simulink model "modificar_acc_compilar"  (R2013b)
settings: Solver=ode45  StartTime=0.0  StopTime=17000  RelTol=1e-3
undefined symbols (not defined in the file): internal_oor, misc_lib, pfb_coeff_gen_calc, xlfda_numerator, xlipgetpartsetting
libraries: xbsIndex_r4 x1539, xps_library x14, dspsigops x8, casper_library_misc x8, casper_library_delays x3, simulink x1
(part 3 of 15)

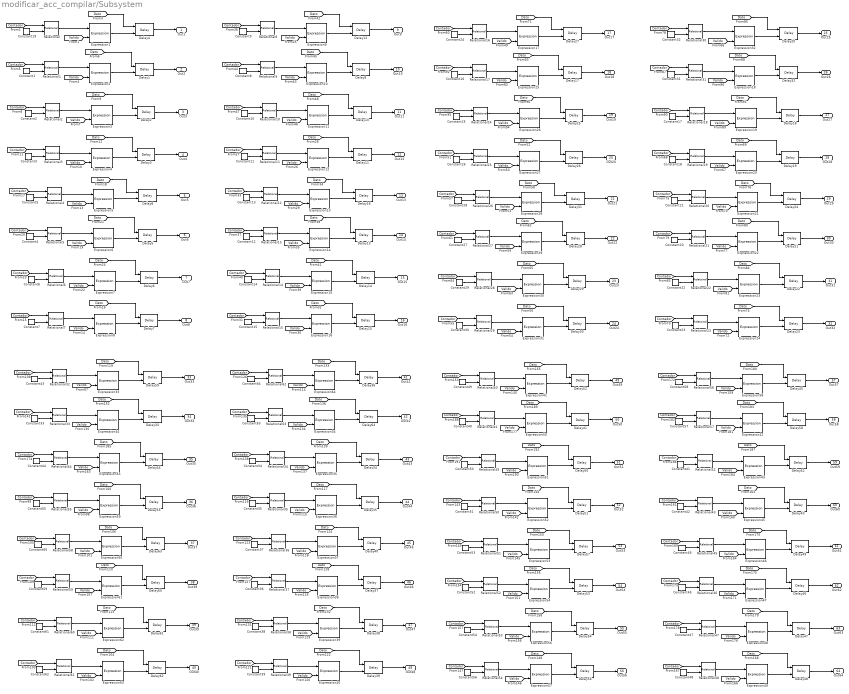
== system modificar_acc_compilar/Subsystem ==
  Constant1 : xbsIndex_r4/Constant  const=1  gui_display_data_type=Fixed-point  arith_type=Unsigned  n_bits=6  bin_pt=0  preci_type=Single  exp_width=8  frac_width=24  explicit_period=on  period=1  equ=P=C  opselect=C  inp2=PCIN>>17  opr=+  inp1=P  carry=CIN  dbl_ovrd=off  block_type=constant
  Constant10 : xbsIndex_r4/Constant  const=10  gui_display_data_type=Fixed-point  arith_type=Unsigned  n_bits=6  bin_pt=0  preci_type=Single  exp_width=8  frac_width=24  explicit_period=on  period=1  equ=P=C  opselect=C  inp2=PCIN>>17  opr=+  inp1=P  carry=CIN  dbl_ovrd=off  block_type=constant
  Constant11 : xbsIndex_r4/Constant  const=11  gui_display_data_type=Fixed-point  arith_type=Unsigned  n_bits=6  bin_pt=0  preci_type=Single  exp_width=8  frac_width=24  explicit_period=on  period=1  equ=P=C  opselect=C  inp2=PCIN>>17  opr=+  inp1=P  carry=CIN  dbl_ovrd=off  block_type=constant
  Constant12 : xbsIndex_r4/Constant  const=13  gui_display_data_type=Fixed-point  arith_type=Unsigned  n_bits=6  bin_pt=0  preci_type=Single  exp_width=8  frac_width=24  explicit_period=on  period=1  equ=P=C  opselect=C  inp2=PCIN>>17  opr=+  inp1=P  carry=CIN  dbl_ovrd=off  block_type=constant
  Constant13 : xbsIndex_r4/Constant  const=12  gui_display_data_type=Fixed-point  arith_type=Unsigned  n_bits=6  bin_pt=0  preci_type=Single  exp_width=8  frac_width=24  explicit_period=on  period=1  equ=P=C  opselect=C  inp2=PCIN>>17  opr=+  inp1=P  carry=CIN  dbl_ovrd=off  block_type=constant
  Constant14 : xbsIndex_r4/Constant  const=14  gui_display_data_type=Fixed-point  arith_type=Unsigned  n_bits=6  bin_pt=0  preci_type=Single  exp_width=8  frac_width=24  explicit_period=on  period=1  equ=P=C  opselect=C  inp2=PCIN>>17  opr=+  inp1=P  carry=CIN  dbl_ovrd=off  block_type=constant
  Constant15 : xbsIndex_r4/Constant  const=15  gui_display_data_type=Fixed-point  arith_type=Unsigned  n_bits=6  bin_pt=0  preci_type=Single  exp_width=8  frac_width=24  explicit_period=on  period=1  equ=P=C  opselect=C  inp2=PCIN>>17  opr=+  inp1=P  carry=CIN  dbl_ovrd=off  block_type=constant
  Constant16 : xbsIndex_r4/Constant  const=17  gui_display_data_type=Fixed-point  arith_type=Unsigned  n_bits=6  bin_pt=0  preci_type=Single  exp_width=8  frac_width=24  explicit_period=on  period=1  equ=P=C  opselect=C  inp2=PCIN>>17  opr=+  inp1=P  carry=CIN  dbl_ovrd=off  block_type=constant
  Constant17 : xbsIndex_r4/Constant  const=26  gui_display_data_type=Fixed-point  arith_type=Unsigned  n_bits=6  bin_pt=0  preci_type=Single  exp_width=8  frac_width=24  explicit_period=on  period=1  equ=P=C  opselect=C  inp2=PCIN>>17  opr=+  inp1=P  carry=CIN  dbl_ovrd=off  block_type=constant
  Constant18 : xbsIndex_r4/Constant  const=27  gui_display_data_type=Fixed-point  arith_type=Unsigned  n_bits=6  bin_pt=0  preci_type=Single  exp_width=8  frac_width=24  explicit_period=on  period=1  equ=P=C  opselect=C  inp2=PCIN>>17  opr=+  inp1=P  carry=CIN  dbl_ovrd=off  block_type=constant
  Constant19 : xbsIndex_r4/Constant  const=0  gui_display_data_type=Fixed-point  arith_type=Unsigned  n_bits=6  bin_pt=0  preci_type=Single  exp_width=8  frac_width=24  explicit_period=on  period=1  equ=P=C  opselect=C  inp2=PCIN>>17  opr=+  inp1=P  carry=CIN  dbl_ovrd=off  block_type=constant
  Constant2 : xbsIndex_r4/Constant  const=2  gui_display_data_type=Fixed-point  arith_type=Unsigned  n_bits=6  bin_pt=0  preci_type=Single  exp_width=8  frac_width=24  explicit_period=on  period=1  equ=P=C  opselect=C  inp2=PCIN>>17  opr=+  inp1=P  carry=CIN  dbl_ovrd=off  block_type=constant
  Constant20 : xbsIndex_r4/Constant  const=29  gui_display_data_type=Fixed-point  arith_type=Unsigned  n_bits=6  bin_pt=0  preci_type=Single  exp_width=8  frac_width=24  explicit_period=on  period=1  equ=P=C  opselect=C  inp2=PCIN>>17  opr=+  inp1=P  carry=CIN  dbl_ovrd=off  block_type=constant
  Constant21 : xbsIndex_r4/Constant  const=28  gui_display_data_type=Fixed-point  arith_type=Unsigned  n_bits=6  bin_pt=0  preci_type=Single  exp_width=8  frac_width=24  explicit_period=on  period=1  equ=P=C  opselect=C  inp2=PCIN>>17  opr=+  inp1=P  carry=CIN  dbl_ovrd=off  block_type=constant
  Constant22 : xbsIndex_r4/Constant  const=30  gui_display_data_type=Fixed-point  arith_type=Unsigned  n_bits=6  bin_pt=0  preci_type=Single  exp_width=8  frac_width=24  explicit_period=on  period=1  equ=P=C  opselect=C  inp2=PCIN>>17  opr=+  inp1=P  carry=CIN  dbl_ovrd=off  block_type=constant
  Constant23 : xbsIndex_r4/Constant  const=31  gui_display_data_type=Fixed-point  arith_type=Unsigned  n_bits=6  bin_pt=0  preci_type=Single  exp_width=8  frac_width=24  explicit_period=on  period=1  equ=P=C  opselect=C  inp2=PCIN>>17  opr=+  inp1=P  carry=CIN  dbl_ovrd=off  block_type=constant
  Constant24 : xbsIndex_r4/Constant  const=16  gui_display_data_type=Fixed-point  arith_type=Unsigned  n_bits=6  bin_pt=0  preci_type=Single  exp_width=8  frac_width=24  explicit_period=on  period=1  equ=P=C  opselect=C  inp2=PCIN>>17  opr=+  inp1=P  carry=CIN  dbl_ovrd=off  block_type=constant
  Constant25 : xbsIndex_r4/Constant  const=18  gui_display_data_type=Fixed-point  arith_type=Unsigned  n_bits=6  bin_pt=0  preci_type=Single  exp_width=8  frac_width=24  explicit_period=on  period=1  equ=P=C  opselect=C  inp2=PCIN>>17  opr=+  inp1=P  carry=CIN  dbl_ovrd=off  block_type=constant
  Constant26 : xbsIndex_r4/Constant  const=19  gui_display_data_type=Fixed-point  arith_type=Unsigned  n_bits=6  bin_pt=0  preci_type=Single  exp_width=8  frac_width=24  explicit_period=on  period=1  equ=P=C  opselect=C  inp2=PCIN>>17  opr=+  inp1=P  carry=CIN  dbl_ovrd=off  block_type=constant
  Constant27 : xbsIndex_r4/Constant  const=21  gui_display_data_type=Fixed-point  arith_type=Unsigned  n_bits=6  bin_pt=0  preci_type=Single  exp_width=8  frac_width=24  explicit_period=on  period=1  equ=P=C  opselect=C  inp2=PCIN>>17  opr=+  inp1=P  carry=CIN  dbl_ovrd=off  block_type=constant
  Constant28 : xbsIndex_r4/Constant  const=20  gui_display_data_type=Fixed-point  arith_type=Unsigned  n_bits=6  bin_pt=0  preci_type=Single  exp_width=8  frac_width=24  explicit_period=on  period=1  equ=P=C  opselect=C  inp2=PCIN>>17  opr=+  inp1=P  carry=CIN  dbl_ovrd=off  block_type=constant
  Constant29 : xbsIndex_r4/Constant  const=22  gui_display_data_type=Fixed-point  arith_type=Unsigned  n_bits=6  bin_pt=0  preci_type=Single  exp_width=8  frac_width=24  explicit_period=on  period=1  equ=P=C  opselect=C  inp2=PCIN>>17  opr=+  inp1=P  carry=CIN  dbl_ovrd=off  block_type=constant
  Constant3 : xbsIndex_r4/Constant  const=3  gui_display_data_type=Fixed-point  arith_type=Unsigned  n_bits=6  bin_pt=0  preci_type=Single  exp_width=8  frac_width=24  explicit_period=on  period=1  equ=P=C  opselect=C  inp2=PCIN>>17  opr=+  inp1=P  carry=CIN  dbl_ovrd=off  block_type=constant
  Constant30 : xbsIndex_r4/Constant  const=23  gui_display_data_type=Fixed-point  arith_type=Unsigned  n_bits=6  bin_pt=0  preci_type=Single  exp_width=8  frac_width=24  explicit_period=on  period=1  equ=P=C  opselect=C  inp2=PCIN>>17  opr=+  inp1=P  carry=CIN  dbl_ovrd=off  block_type=constant
  Constant31 : xbsIndex_r4/Constant  const=25  gui_display_data_type=Fixed-point  arith_type=Unsigned  n_bits=6  bin_pt=0  preci_type=Single  exp_width=8  frac_width=24  explicit_period=on  period=1  equ=P=C  opselect=C  inp2=PCIN>>17  opr=+  inp1=P  carry=CIN  dbl_ovrd=off  block_type=constant
  Constant32 : xbsIndex_r4/Constant  const=24  gui_display_data_type=Fixed-point  arith_type=Unsigned  n_bits=6  bin_pt=0  preci_type=Single  exp_width=8  frac_width=24  explicit_period=on  period=1  equ=P=C  opselect=C  inp2=PCIN>>17  opr=+  inp1=P  carry=CIN  dbl_ovrd=off  block_type=constant
  Constant33 : xbsIndex_r4/Constant  const=33  gui_display_data_type=Fixed-point  arith_type=Unsigned  n_bits=6  bin_pt=0  preci_type=Single  exp_width=8  frac_width=24  explicit_period=on  period=1  equ=P=C  opselect=C  inp2=PCIN>>17  opr=+  inp1=P  carry=CIN  dbl_ovrd=off  block_type=constant
  Constant34 : xbsIndex_r4/Constant  const=42  gui_display_data_type=Fixed-point  arith_type=Unsigned  n_bits=6  bin_pt=0  preci_type=Single  exp_width=8  frac_width=24  explicit_period=on  period=1  equ=P=C  opselect=C  inp2=PCIN>>17  opr=+  inp1=P  carry=CIN  dbl_ovrd=off  block_type=constant
  Constant35 : xbsIndex_r4/Constant  const=43  gui_display_data_type=Fixed-point  arith_type=Unsigned  n_bits=6  bin_pt=0  preci_type=Single  exp_width=8  frac_width=24  explicit_period=on  period=1  equ=P=C  opselect=C  inp2=PCIN>>17  opr=+  inp1=P  carry=CIN  dbl_ovrd=off  block_type=constant
  Constant36 : xbsIndex_r4/Constant  const=45  gui_display_data_type=Fixed-point  arith_type=Unsigned  n_bits=6  bin_pt=0  preci_type=Single  exp_width=8  frac_width=24  explicit_period=on  period=1  equ=P=C  opselect=C  inp2=PCIN>>17  opr=+  inp1=P  carry=CIN  dbl_ovrd=off  block_type=constant
  Constant37 : xbsIndex_r4/Constant  const=44  gui_display_data_type=Fixed-point  arith_type=Unsigned  n_bits=6  bin_pt=0  preci_type=Single  exp_width=8  frac_width=24  explicit_period=on  period=1  equ=P=C  opselect=C  inp2=PCIN>>17  opr=+  inp1=P  carry=CIN  dbl_ovrd=off  block_type=constant
  Constant38 : xbsIndex_r4/Constant  const=46  gui_display_data_type=Fixed-point  arith_type=Unsigned  n_bits=6  bin_pt=0  preci_type=Single  exp_width=8  frac_width=24  explicit_period=on  period=1  equ=P=C  opselect=C  inp2=PCIN>>17  opr=+  inp1=P  carry=CIN  dbl_ovrd=off  block_type=constant
  Constant39 : xbsIndex_r4/Constant  const=47  gui_display_data_type=Fixed-point  arith_type=Unsigned  n_bits=6  bin_pt=0  preci_type=Single  exp_width=8  frac_width=24  explicit_period=on  period=1  equ=P=C  opselect=C  inp2=PCIN>>17  opr=+  inp1=P  carry=CIN  dbl_ovrd=off  block_type=constant
  Constant4 : xbsIndex_r4/Constant  const=5  gui_display_data_type=Fixed-point  arith_type=Unsigned  n_bits=6  bin_pt=0  preci_type=Single  exp_width=8  frac_width=24  explicit_period=on  period=1  equ=P=C  opselect=C  inp2=PCIN>>17  opr=+  inp1=P  carry=CIN  dbl_ovrd=off  block_type=constant
  Constant40 : xbsIndex_r4/Constant  const=49  gui_display_data_type=Fixed-point  arith_type=Unsigned  n_bits=6  bin_pt=0  preci_type=Single  exp_width=8  frac_width=24  explicit_period=on  period=1  equ=P=C  opselect=C  inp2=PCIN>>17  opr=+  inp1=P  carry=CIN  dbl_ovrd=off  block_type=constant
  Constant41 : xbsIndex_r4/Constant  const=58  gui_display_data_type=Fixed-point  arith_type=Unsigned  n_bits=6  bin_pt=0  preci_type=Single  exp_width=8  frac_width=24  explicit_period=on  period=1  equ=P=C  opselect=C  inp2=PCIN>>17  opr=+  inp1=P  carry=CIN  dbl_ovrd=off  block_type=constant
  Constant42 : xbsIndex_r4/Constant  const=59  gui_display_data_type=Fixed-point  arith_type=Unsigned  n_bits=6  bin_pt=0  preci_type=Single  exp_width=8  frac_width=24  explicit_period=on  period=1  equ=P=C  opselect=C  inp2=PCIN>>17  opr=+  inp1=P  carry=CIN  dbl_ovrd=off  block_type=constant
  Constant43 : xbsIndex_r4/Constant  const=32  gui_display_data_type=Fixed-point  arith_type=Unsigned  n_bits=6  bin_pt=0  preci_type=Single  exp_width=8  frac_width=24  explicit_period=on  period=1  equ=P=C  opselect=C  inp2=PCIN>>17  opr=+  inp1=P  carry=CIN  dbl_ovrd=off  block_type=constant
  Constant44 : xbsIndex_r4/Constant  const=34  gui_display_data_type=Fixed-point  arith_type=Unsigned  n_bits=6  bin_pt=0  preci_type=Single  exp_width=8  frac_width=24  explicit_period=on  period=1  equ=P=C  opselect=C  inp2=PCIN>>17  opr=+  inp1=P  carry=CIN  dbl_ovrd=off  block_type=constant
  Constant45 : xbsIndex_r4/Constant  const=61  gui_display_data_type=Fixed-point  arith_type=Unsigned  n_bits=6  bin_pt=0  preci_type=Single  exp_width=8  frac_width=24  explicit_period=on  period=1  equ=P=C  opselect=C  inp2=PCIN>>17  opr=+  inp1=P  carry=CIN  dbl_ovrd=off  block_type=constant
  Constant46 : xbsIndex_r4/Constant  const=60  gui_display_data_type=Fixed-point  arith_type=Unsigned  n_bits=6  bin_pt=0  preci_type=Single  exp_width=8  frac_width=24  explicit_period=on  period=1  equ=P=C  opselect=C  inp2=PCIN>>17  opr=+  inp1=P  carry=CIN  dbl_ovrd=off  block_type=constant
  Constant47 : xbsIndex_r4/Constant  const=62  gui_display_data_type=Fixed-point  arith_type=Unsigned  n_bits=6  bin_pt=0  preci_type=Single  exp_width=8  frac_width=24  explicit_period=on  period=1  equ=P=C  opselect=C  inp2=PCIN>>17  opr=+  inp1=P  carry=CIN  dbl_ovrd=off  block_type=constant
  Constant48 : xbsIndex_r4/Constant  const=63  gui_display_data_type=Fixed-point  arith_type=Unsigned  n_bits=6  bin_pt=0  preci_type=Single  exp_width=8  frac_width=24  explicit_period=on  period=1  equ=P=C  opselect=C  inp2=PCIN>>17  opr=+  inp1=P  carry=CIN  dbl_ovrd=off  block_type=constant
  Constant49 : xbsIndex_r4/Constant  const=48  gui_display_data_type=Fixed-point  arith_type=Unsigned  n_bits=6  bin_pt=0  preci_type=Single  exp_width=8  frac_width=24  explicit_period=on  period=1  equ=P=C  opselect=C  inp2=PCIN>>17  opr=+  inp1=P  carry=CIN  dbl_ovrd=off  block_type=constant
  Constant5 : xbsIndex_r4/Constant  const=4  gui_display_data_type=Fixed-point  arith_type=Unsigned  n_bits=6  bin_pt=0  preci_type=Single  exp_width=8  frac_width=24  explicit_period=on  period=1  equ=P=C  opselect=C  inp2=PCIN>>17  opr=+  inp1=P  carry=CIN  dbl_ovrd=off  block_type=constant
  Constant50 : xbsIndex_r4/Constant  const=50  gui_display_data_type=Fixed-point  arith_type=Unsigned  n_bits=6  bin_pt=0  preci_type=Single  exp_width=8  frac_width=24  explicit_period=on  period=1  equ=P=C  opselect=C  inp2=PCIN>>17  opr=+  inp1=P  carry=CIN  dbl_ovrd=off  block_type=constant
  Constant51 : xbsIndex_r4/Constant  const=51  gui_display_data_type=Fixed-point  arith_type=Unsigned  n_bits=6  bin_pt=0  preci_type=Single  exp_width=8  frac_width=24  explicit_period=on  period=1  equ=P=C  opselect=C  inp2=PCIN>>17  opr=+  inp1=P  carry=CIN  dbl_ovrd=off  block_type=constant
  Constant52 : xbsIndex_r4/Constant  const=53  gui_display_data_type=Fixed-point  arith_type=Unsigned  n_bits=6  bin_pt=0  preci_type=Single  exp_width=8  frac_width=24  explicit_period=on  period=1  equ=P=C  opselect=C  inp2=PCIN>>17  opr=+  inp1=P  carry=CIN  dbl_ovrd=off  block_type=constant
  Constant53 : xbsIndex_r4/Constant  const=52  gui_display_data_type=Fixed-point  arith_type=Unsigned  n_bits=6  bin_pt=0  preci_type=Single  exp_width=8  frac_width=24  explicit_period=on  period=1  equ=P=C  opselect=C  inp2=PCIN>>17  opr=+  inp1=P  carry=CIN  dbl_ovrd=off  block_type=constant
  Constant54 : xbsIndex_r4/Constant  const=54  gui_display_data_type=Fixed-point  arith_type=Unsigned  n_bits=6  bin_pt=0  preci_type=Single  exp_width=8  frac_width=24  explicit_period=on  period=1  equ=P=C  opselect=C  inp2=PCIN>>17  opr=+  inp1=P  carry=CIN  dbl_ovrd=off  block_type=constant
  Constant55 : xbsIndex_r4/Constant  const=35  gui_display_data_type=Fixed-point  arith_type=Unsigned  n_bits=6  bin_pt=0  preci_type=Single  exp_width=8  frac_width=24  explicit_period=on  period=1  equ=P=C  opselect=C  inp2=PCIN>>17  opr=+  inp1=P  carry=CIN  dbl_ovrd=off  block_type=constant
  Constant56 : xbsIndex_r4/Constant  const=55  gui_display_data_type=Fixed-point  arith_type=Unsigned  n_bits=6  bin_pt=0  preci_type=Single  exp_width=8  frac_width=24  explicit_period=on  period=1  equ=P=C  opselect=C  inp2=PCIN>>17  opr=+  inp1=P  carry=CIN  dbl_ovrd=off  block_type=constant
  Constant57 : xbsIndex_r4/Constant  const=57  gui_display_data_type=Fixed-point  arith_type=Unsigned  n_bits=6  bin_pt=0  preci_type=Single  exp_width=8  frac_width=24  explicit_period=on  period=1  equ=P=C  opselect=C  inp2=PCIN>>17  opr=+  inp1=P  carry=CIN  dbl_ovrd=off  block_type=constant
  Constant58 : xbsIndex_r4/Constant  const=56  gui_display_data_type=Fixed-point  arith_type=Unsigned  n_bits=6  bin_pt=0  preci_type=Single  exp_width=8  frac_width=24  explicit_period=on  period=1  equ=P=C  opselect=C  inp2=PCIN>>17  opr=+  inp1=P  carry=CIN  dbl_ovrd=off  block_type=constant
  Constant59 : xbsIndex_r4/Constant  const=37  gui_display_data_type=Fixed-point  arith_type=Unsigned  n_bits=6  bin_pt=0  preci_type=Single  exp_width=8  frac_width=24  explicit_period=on  period=1  equ=P=C  opselect=C  inp2=PCIN>>17  opr=+  inp1=P  carry=CIN  dbl_ovrd=off  block_type=constant
  Constant6 : xbsIndex_r4/Constant  const=6  gui_display_data_type=Fixed-point  arith_type=Unsigned  n_bits=6  bin_pt=0  preci_type=Single  exp_width=8  frac_width=24  explicit_period=on  period=1  equ=P=C  opselect=C  inp2=PCIN>>17  opr=+  inp1=P  carry=CIN  dbl_ovrd=off  block_type=constant
  Constant60 : xbsIndex_r4/Constant  const=36  gui_display_data_type=Fixed-point  arith_type=Unsigned  n_bits=6  bin_pt=0  preci_type=Single  exp_width=8  frac_width=24  explicit_period=on  period=1  equ=P=C  opselect=C  inp2=PCIN>>17  opr=+  inp1=P  carry=CIN  dbl_ovrd=off  block_type=constant
  Constant61 : xbsIndex_r4/Constant  const=38  gui_display_data_type=Fixed-point  arith_type=Unsigned  n_bits=6  bin_pt=0  preci_type=Single  exp_width=8  frac_width=24  explicit_period=on  period=1  equ=P=C  opselect=C  inp2=PCIN>>17  opr=+  inp1=P  carry=CIN  dbl_ovrd=off  block_type=constant
  Constant62 : xbsIndex_r4/Constant  const=39  gui_display_data_type=Fixed-point  arith_type=Unsigned  n_bits=6  bin_pt=0  preci_type=Single  exp_width=8  frac_width=24  explicit_period=on  period=1  equ=P=C  opselect=C  inp2=PCIN>>17  opr=+  inp1=P  carry=CIN  dbl_ovrd=off  block_type=constant
  Constant63 : xbsIndex_r4/Constant  const=41  gui_display_data_type=Fixed-point  arith_type=Unsigned  n_bits=6  bin_pt=0  preci_type=Single  exp_width=8  frac_width=24  explicit_period=on  period=1  equ=P=C  opselect=C  inp2=PCIN>>17  opr=+  inp1=P  carry=CIN  dbl_ovrd=off  block_type=constant
  Constant64 : xbsIndex_r4/Constant  const=40  gui_display_data_type=Fixed-point  arith_type=Unsigned  n_bits=6  bin_pt=0  preci_type=Single  exp_width=8  frac_width=24  explicit_period=on  period=1  equ=P=C  opselect=C  inp2=PCIN>>17  opr=+  inp1=P  carry=CIN  dbl_ovrd=off  block_type=constant
  Constant7 : xbsIndex_r4/Constant  const=7  gui_display_data_type=Fixed-point  arith_type=Unsigned  n_bits=6  bin_pt=0  preci_type=Single  exp_width=8  frac_width=24  explicit_period=on  period=1  equ=P=C  opselect=C  inp2=PCIN>>17  opr=+  inp1=P  carry=CIN  dbl_ovrd=off  block_type=constant
  Constant8 : xbsIndex_r4/Constant  const=9  gui_display_data_type=Fixed-point  arith_type=Unsigned  n_bits=6  bin_pt=0  preci_type=Single  exp_width=8  frac_width=24  explicit_period=on  period=1  equ=P=C  opselect=C  inp2=PCIN>>17  opr=+  inp1=P  carry=CIN  dbl_ovrd=off  block_type=constant
  Constant9 : xbsIndex_r4/Constant  const=8  gui_display_data_type=Fixed-point  arith_type=Unsigned  n_bits=6  bin_pt=0  preci_type=Single  exp_width=8  frac_width=24  explicit_period=on  period=1  equ=P=C  opselect=C  inp2=PCIN>>17  opr=+  inp1=P  carry=CIN  dbl_ovrd=off  block_type=constant
  Delay1 : xbsIndex_r4/Delay  rst=off  infoeditControl=Selection of Reset will increase slice count due to use of real FFs and instead of SRLs  en=on  latency=2  dbl_ovrd=off  reg_retiming=off  block_type=delay
      settings: xl_area=[24 48 0 48 0 0 0]
  Delay10 : xbsIndex_r4/Delay  rst=off  infoeditControl=Selection of Reset will increase slice count due to use of real FFs and instead of SRLs  en=on  latency=11  dbl_ovrd=off  reg_retiming=off  block_type=delay
      settings: xl_area=[24 48 0 48 0 0 0]
  Delay11 : xbsIndex_r4/Delay  rst=off  infoeditControl=Selection of Reset will increase slice count due to use of real FFs and instead of SRLs  en=on  latency=12  dbl_ovrd=off  reg_retiming=off  block_type=delay
      settings: xl_area=[24 48 0 48 0 0 0]
  Delay12 : xbsIndex_r4/Delay  rst=off  infoeditControl=Selection of Reset will increase slice count due to use of real FFs and instead of SRLs  en=on  latency=9  dbl_ovrd=off  reg_retiming=off  block_type=delay
      settings: xl_area=[24 48 0 48 0 0 0]
  Delay13 : xbsIndex_r4/Delay  rst=off  infoeditControl=Selection of Reset will increase slice count due to use of real FFs and instead of SRLs  en=on  latency=14  dbl_ovrd=off  reg_retiming=off  block_type=delay
      settings: xl_area=[18 36 0 36 0 0 0]
  Delay14 : xbsIndex_r4/Delay  rst=off  infoeditControl=Selection of Reset will increase slice count due to use of real FFs and instead of SRLs  en=on  latency=15  dbl_ovrd=off  reg_retiming=off  block_type=delay
      settings: xl_area=[18 36 0 36 0 0 0]
  Delay15 : xbsIndex_r4/Delay  rst=off  infoeditControl=Selection of Reset will increase slice count due to use of real FFs and instead of SRLs  en=on  latency=16  dbl_ovrd=off  reg_retiming=off  block_type=delay
      settings: xl_area=[18 36 0 36 0 0 0]
  Delay16 : xbsIndex_r4/Delay  rst=off  infoeditControl=Selection of Reset will increase slice count due to use of real FFs and instead of SRLs  en=on  latency=13  dbl_ovrd=off  reg_retiming=off  block_type=delay
      settings: xl_area=[24 48 0 36 0 0 0]
  Delay17 : xbsIndex_r4/Delay  rst=off  infoeditControl=Selection of Reset will increase slice count due to use of real FFs and instead of SRLs  en=on  latency=18  dbl_ovrd=off  reg_retiming=off  block_type=delay
      settings: xl_area=[18 36 0 36 0 0 0]
  Delay18 : xbsIndex_r4/Delay  rst=off  infoeditControl=Selection of Reset will increase slice count due to use of real FFs and instead of SRLs  en=on  latency=27  dbl_ovrd=off  reg_retiming=off  block_type=delay
      settings: xl_area=[18 36 0 36 0 0 0]
  Delay19 : xbsIndex_r4/Delay  rst=off  infoeditControl=Selection of Reset will increase slice count due to use of real FFs and instead of SRLs  en=on  latency=28  dbl_ovrd=off  reg_retiming=off  block_type=delay
      settings: xl_area=[18 36 0 36 0 0 0]
  Delay2 : xbsIndex_r4/Delay  rst=off  infoeditControl=Selection of Reset will increase slice count due to use of real FFs and instead of SRLs  en=on  latency=3  dbl_ovrd=off  reg_retiming=off  block_type=delay
      settings: xl_area=[24 48 0 48 0 0 0]
  Delay20 : xbsIndex_r4/Delay  rst=off  infoeditControl=Selection of Reset will increase slice count due to use of real FFs and instead of SRLs  en=on  latency=25  dbl_ovrd=off  reg_retiming=off  block_type=delay
      settings: xl_area=[18 36 0 36 0 0 0]
  Delay21 : xbsIndex_r4/Delay  rst=off  infoeditControl=Selection of Reset will increase slice count due to use of real FFs and instead of SRLs  en=on  latency=30  dbl_ovrd=off  reg_retiming=off  block_type=delay
      settings: xl_area=[18 36 0 24 0 0 0]
  Delay22 : xbsIndex_r4/Delay  rst=off  infoeditControl=Selection of Reset will increase slice count due to use of real FFs and instead of SRLs  en=on  latency=31  dbl_ovrd=off  reg_retiming=off  block_type=delay
      settings: xl_area=[12 24 0 24 0 0 0]
  Delay23 : xbsIndex_r4/Delay  rst=off  infoeditControl=Selection of Reset will increase slice count due to use of real FFs and instead of SRLs  en=on  latency=32  dbl_ovrd=off  reg_retiming=off  block_type=delay
      settings: xl_area=[12 24 0 24 0 0 0]
  Delay24 : xbsIndex_r4/Delay  rst=off  infoeditControl=Selection of Reset will increase slice count due to use of real FFs and instead of SRLs  en=on  latency=29  dbl_ovrd=off  reg_retiming=off  block_type=delay
      settings: xl_area=[18 36 0 36 0 0 0]
  Delay25 : xbsIndex_r4/Delay  rst=off  infoeditControl=Selection of Reset will increase slice count due to use of real FFs and instead of SRLs  en=on  latency=19  dbl_ovrd=off  reg_retiming=off  block_type=delay
      settings: xl_area=[18 36 0 36 0 0 0]
  Delay26 : xbsIndex_r4/Delay  rst=off  infoeditControl=Selection of Reset will increase slice count due to use of real FFs and instead of SRLs  en=on  latency=20  dbl_ovrd=off  reg_retiming=off  block_type=delay
      settings: xl_area=[18 36 0 36 0 0 0]
  Delay27 : xbsIndex_r4/Delay  rst=off  infoeditControl=Selection of Reset will increase slice count due to use of real FFs and instead of SRLs  en=on  latency=17  dbl_ovrd=off  reg_retiming=off  block_type=delay
      settings: xl_area=[18 36 0 36 0 0 0]
  Delay28 : xbsIndex_r4/Delay  rst=off  infoeditControl=Selection of Reset will increase slice count due to use of real FFs and instead of SRLs  en=on  latency=22  dbl_ovrd=off  reg_retiming=off  block_type=delay
      settings: xl_area=[18 36 0 36 0 0 0]
  Delay29 : xbsIndex_r4/Delay  rst=off  infoeditControl=Selection of Reset will increase slice count due to use of real FFs and instead of SRLs  en=on  latency=23  dbl_ovrd=off  reg_retiming=off  block_type=delay
      settings: xl_area=[18 36 0 36 0 0 0]
  Delay3 : xbsIndex_r4/Delay  rst=off  infoeditControl=Selection of Reset will increase slice count due to use of real FFs and instead of SRLs  en=on  latency=4  dbl_ovrd=off  reg_retiming=off  block_type=delay
      settings: xl_area=[24 48 0 48 0 0 0]
  Delay30 : xbsIndex_r4/Delay  rst=off  infoeditControl=Selection of Reset will increase slice count due to use of real FFs and instead of SRLs  en=on  latency=24  dbl_ovrd=off  reg_retiming=off  block_type=delay
      settings: xl_area=[18 36 0 36 0 0 0]
  Delay31 : xbsIndex_r4/Delay  rst=off  infoeditControl=Selection of Reset will increase slice count due to use of real FFs and instead of SRLs  en=on  latency=21  dbl_ovrd=off  reg_retiming=off  block_type=delay
      settings: xl_area=[18 36 0 36 0 0 0]
  Delay32 : xbsIndex_r4/Delay  rst=off  infoeditControl=Selection of Reset will increase slice count due to use of real FFs and instead of SRLs  en=on  latency=26  dbl_ovrd=off  reg_retiming=off  block_type=delay
      settings: xl_area=[18 36 0 36 0 0 0]
  Delay33 : xbsIndex_r4/Delay  rst=off  infoeditControl=Selection of Reset will increase slice count due to use of real FFs and instead of SRLs  en=on  latency=34  dbl_ovrd=off  reg_retiming=off  block_type=delay
      settings: xl_area=[12 24 0 24 0 0 0]
  Delay34 : xbsIndex_r4/Delay  rst=off  infoeditControl=Selection of Reset will increase slice count due to use of real FFs and instead of SRLs  en=on  latency=43  dbl_ovrd=off  reg_retiming=off  block_type=delay
      settings: xl_area=[12 24 0 24 0 0 0]
  Delay35 : xbsIndex_r4/Delay  rst=off  infoeditControl=Selection of Reset will increase slice count due to use of real FFs and instead of SRLs  en=on  latency=44  dbl_ovrd=off  reg_retiming=off  block_type=delay
      settings: xl_area=[12 24 0 24 0 0 0]
  Delay36 : xbsIndex_r4/Delay  rst=off  infoeditControl=Selection of Reset will increase slice count due to use of real FFs and instead of SRLs  en=on  latency=41  dbl_ovrd=off  reg_retiming=off  block_type=delay
      settings: xl_area=[12 24 0 24 0 0 0]
  Delay37 : xbsIndex_r4/Delay  rst=off  infoeditControl=Selection of Reset will increase slice count due to use of real FFs and instead of SRLs  en=on  latency=46  dbl_ovrd=off  reg_retiming=off  block_type=delay
      settings: xl_area=[12 24 0 24 0 0 0]
  Delay38 : xbsIndex_r4/Delay  rst=off  infoeditControl=Selection of Reset will increase slice count due to use of real FFs and instead of SRLs  en=on  latency=47  dbl_ovrd=off  reg_retiming=off  block_type=delay
      settings: xl_area=[12 24 0 12 0 0 0]
  Delay39 : xbsIndex_r4/Delay  rst=off  infoeditControl=Selection of Reset will increase slice count due to use of real FFs and instead of SRLs  en=on  latency=48  dbl_ovrd=off  reg_retiming=off  block_type=delay
      settings: xl_area=[6 12 0 12 0 0 0]
  Delay4 : xbsIndex_r4/Delay  rst=off  infoeditControl=Selection of Reset will increase slice count due to use of real FFs and instead of SRLs  en=on  latency=1  dbl_ovrd=off  reg_retiming=off  block_type=delay
      settings: xl_area=[24 48 0 48 0 0 0]
  Delay40 : xbsIndex_r4/Delay  rst=off  infoeditControl=Selection of Reset will increase slice count due to use of real FFs and instead of SRLs  en=on  latency=45  dbl_ovrd=off  reg_retiming=off  block_type=delay
      settings: xl_area=[12 24 0 24 0 0 0]
  Delay41 : xbsIndex_r4/Delay  rst=off  infoeditControl=Selection of Reset will increase slice count due to use of real FFs and instead of SRLs  en=on  latency=50  dbl_ovrd=off  reg_retiming=off  block_type=delay
      settings: xl_area=[6 12 0 12 0 0 0]
  Delay42 : xbsIndex_r4/Delay  rst=off  infoeditControl=Selection of Reset will increase slice count due to use of real FFs and instead of SRLs  en=on  latency=59  dbl_ovrd=off  reg_retiming=off  block_type=delay
      settings: xl_area=[6 12 0 12 0 0 0]
  Delay43 : xbsIndex_r4/Delay  rst=off  infoeditControl=Selection of Reset will increase slice count due to use of real FFs and instead of SRLs  en=on  latency=60  dbl_ovrd=off  reg_retiming=off  block_type=delay
      settings: xl_area=[6 12 0 12 0 0 0]
  Delay44 : xbsIndex_r4/Delay  rst=off  infoeditControl=Selection of Reset will increase slice count due to use of real FFs and instead of SRLs  en=on  latency=35  dbl_ovrd=off  reg_retiming=off  block_type=delay
      settings: xl_area=[12 24 0 24 0 0 0]
  Delay45 : xbsIndex_r4/Delay  rst=off  infoeditControl=Selection of Reset will increase slice count due to use of real FFs and instead of SRLs  en=on  latency=57  dbl_ovrd=off  reg_retiming=off  block_type=delay
      settings: xl_area=[6 12 0 12 0 0 0]
  Delay46 : xbsIndex_r4/Delay  rst=off  infoeditControl=Selection of Reset will increase slice count due to use of real FFs and instead of SRLs  en=on  latency=62  dbl_ovrd=off  reg_retiming=off  block_type=delay
      settings: xl_area=[6 12 0 12 0 0 0]
  Delay47 : xbsIndex_r4/Delay  rst=off  infoeditControl=Selection of Reset will increase slice count due to use of real FFs and instead of SRLs  en=on  latency=63  dbl_ovrd=off  reg_retiming=off  block_type=delay
      settings: xl_area=[6 12 0 12 0 0 0]
  Delay48 : xbsIndex_r4/Delay  rst=off  infoeditControl=Selection of Reset will increase slice count due to use of real FFs and instead of SRLs  en=on  latency=64  dbl_ovrd=off  reg_retiming=off  block_type=delay
      settings: xl_area=[6 12 0 0 0 0 0]
  Delay49 : xbsIndex_r4/Delay  rst=off  infoeditControl=Selection of Reset will increase slice count due to use of real FFs and instead of SRLs  en=on  latency=61  dbl_ovrd=off  reg_retiming=off  block_type=delay
      settings: xl_area=[6 12 0 12 0 0 0]
  Delay5 : xbsIndex_r4/Delay  rst=off  infoeditControl=Selection of Reset will increase slice count due to use of real FFs and instead of SRLs  en=on  latency=6  dbl_ovrd=off  reg_retiming=off  block_type=delay
      settings: xl_area=[24 48 0 48 0 0 0]
  Delay50 : xbsIndex_r4/Delay  rst=off  infoeditControl=Selection of Reset will increase slice count due to use of real FFs and instead of SRLs  en=on  latency=51  dbl_ovrd=off  reg_retiming=off  block_type=delay
      settings: xl_area=[6 12 0 12 0 0 0]
  Delay51 : xbsIndex_r4/Delay  rst=off  infoeditControl=Selection of Reset will increase slice count due to use of real FFs and instead of SRLs  en=on  latency=52  dbl_ovrd=off  reg_retiming=off  block_type=delay
      settings: xl_area=[6 12 0 12 0 0 0]
  Delay52 : xbsIndex_r4/Delay  rst=off  infoeditControl=Selection of Reset will increase slice count due to use of real FFs and instead of SRLs  en=on  latency=49  dbl_ovrd=off  reg_retiming=off  block_type=delay
      settings: xl_area=[6 12 0 12 0 0 0]
  Delay53 : xbsIndex_r4/Delay  rst=off  infoeditControl=Selection of Reset will increase slice count due to use of real FFs and instead of SRLs  en=on  latency=54  dbl_ovrd=off  reg_retiming=off  block_type=delay
      settings: xl_area=[6 12 0 12 0 0 0]
  Delay54 : xbsIndex_r4/Delay  rst=off  infoeditControl=Selection of Reset will increase slice count due to use of real FFs and instead of SRLs  en=on  latency=55  dbl_ovrd=off  reg_retiming=off  block_type=delay
      settings: xl_area=[6 12 0 12 0 0 0]
  Delay55 : xbsIndex_r4/Delay  rst=off  infoeditControl=Selection of Reset will increase slice count due to use of real FFs and instead of SRLs  en=on  latency=36  dbl_ovrd=off  reg_retiming=off  block_type=delay
      settings: xl_area=[12 24 0 24 0 0 0]
  Delay56 : xbsIndex_r4/Delay  rst=off  infoeditControl=Selection of Reset will increase slice count due to use of real FFs and instead of SRLs  en=on  latency=56  dbl_ovrd=off  reg_retiming=off  block_type=delay
      settings: xl_area=[6 12 0 12 0 0 0]
  Delay57 : xbsIndex_r4/Delay  rst=off  infoeditControl=Selection of Reset will increase slice count due to use of real FFs and instead of SRLs  en=on  latency=53  dbl_ovrd=off  reg_retiming=off  block_type=delay
      settings: xl_area=[6 12 0 12 0 0 0]
  Delay58 : xbsIndex_r4/Delay  rst=off  infoeditControl=Selection of Reset will increase slice count due to use of real FFs and instead of SRLs  en=on  latency=58  dbl_ovrd=off  reg_retiming=off  block_type=delay
      settings: xl_area=[6 12 0 12 0 0 0]
  Delay59 : xbsIndex_r4/Delay  rst=off  infoeditControl=Selection of Reset will increase slice count due to use of real FFs and instead of SRLs  en=on  latency=33  dbl_ovrd=off  reg_retiming=off  block_type=delay
      settings: xl_area=[12 24 0 24 0 0 0]
  Delay6 : xbsIndex_r4/Delay  rst=off  infoeditControl=Selection of Reset will increase slice count due to use of real FFs and instead of SRLs  en=on  latency=7  dbl_ovrd=off  reg_retiming=off  block_type=delay
      settings: xl_area=[24 48 0 48 0 0 0]
  Delay60 : xbsIndex_r4/Delay  rst=off  infoeditControl=Selection of Reset will increase slice count due to use of real FFs and instead of SRLs  en=on  latency=38  dbl_ovrd=off  reg_retiming=off  block_type=delay
      settings: xl_area=[12 24 0 24 0 0 0]
  Delay61 : xbsIndex_r4/Delay  rst=off  infoeditControl=Selection of Reset will increase slice count due to use of real FFs and instead of SRLs  en=on  latency=39  dbl_ovrd=off  reg_retiming=off  block_type=delay
      settings: xl_area=[12 24 0 24 0 0 0]
  Delay62 : xbsIndex_r4/Delay  rst=off  infoeditControl=Selection of Reset will increase slice count due to use of real FFs and instead of SRLs  en=on  latency=40  dbl_ovrd=off  reg_retiming=off  block_type=delay
      settings: xl_area=[12 24 0 24 0 0 0]
  Delay63 : xbsIndex_r4/Delay  rst=off  infoeditControl=Selection of Reset will increase slice count due to use of real FFs and instead of SRLs  en=on  latency=37  dbl_ovrd=off  reg_retiming=off  block_type=delay
      settings: xl_area=[12 24 0 24 0 0 0]
  Delay64 : xbsIndex_r4/Delay  rst=off  infoeditControl=Selection of Reset will increase slice count due to use of real FFs and instead of SRLs  en=on  latency=42  dbl_ovrd=off  reg_retiming=off  block_type=delay
      settings: xl_area=[12 24 0 24 0 0 0]
  Delay7 : xbsIndex_r4/Delay  rst=off  infoeditControl=Selection of Reset will increase slice count due to use of real FFs and instead of SRLs  en=on  latency=8  dbl_ovrd=off  reg_retiming=off  block_type=delay
      settings: xl_area=[24 48 0 48 0 0 0]
  Delay8 : xbsIndex_r4/Delay  rst=off  infoeditControl=Selection of Reset will increase slice count due to use of real FFs and instead of SRLs  en=on  latency=5  dbl_ovrd=off  reg_retiming=off  block_type=delay
      settings: xl_area=[24 48 0 48 0 0 0]
  Delay9 : xbsIndex_r4/Delay  rst=off  infoeditControl=Selection of Reset will increase slice count due to use of real FFs and instead of SRLs  en=on  latency=10  dbl_ovrd=off  reg_retiming=off  block_type=delay
      settings: xl_area=[24 48 0 48 0 0 0]
  Expression{1..64} (64 alike) : xbsIndex_r4/Expression  expression=a & b  align_bp=on  en=off  latency=0  precision=Full  arith_type=Unsigned  n_bits=16  bin_pt=0  dbl_ovrd=off  block_type=expr
  Relational{,1..63} (64 alike) : xbsIndex_r4/Relational  mode=a=b  en=off  latency=0  dbl_ovrd=off  block_type=relational
      settings: xl_area=[2 0 0 3 0 0 0]
  Out1 : Outport
  Out2 : Outport  Port=2
  Out3 : Outport  Port=3
  Out4 : Outport  Port=4
  Out5 : Outport  Port=5
  Out6 : Outport  Port=6
  Out7 : Outport  Port=7
  Out8 : Outport  Port=8
  Out9 : Outport  Port=9
  Out10 : Outport  Port=10
  Out11 : Outport  Port=11
  Out12 : Outport  Port=12
  Out13 : Outport  Port=13
  Out14 : Outport  Port=14
  Out15 : Outport  Port=15
  Out16 : Outport  Port=16
  Out17 : Outport  Port=17
  Out18 : Outport  Port=18
  Out19 : Outport  Port=19
  Out20 : Outport  Port=20
  Out21 : Outport  Port=21
  Out22 : Outport  Port=22
  Out23 : Outport  Port=23
  Out24 : Outport  Port=24
  Out25 : Outport  Port=25
  Out26 : Outport  Port=26
  Out27 : Outport  Port=27
  Out28 : Outport  Port=28
  Out29 : Outport  Port=29
  Out30 : Outport  Port=30
  Out31 : Outport  Port=31
  Out32 : Outport  Port=32
  Out33 : Outport  Port=33
  Out34 : Outport  Port=34
  Out35 : Outport  Port=35
  Out36 : Outport  Port=36
  Out37 : Outport  Port=37
  Out38 : Outport  Port=38
  Out39 : Outport  Port=39
  Out40 : Outport  Port=40
  Out41 : Outport  Port=41
  Out42 : Outport  Port=42
  Out43 : Outport  Port=43
  Out44 : Outport  Port=44
  Out45 : Outport  Port=45
  Out46 : Outport  Port=46
  Out47 : Outport  Port=47
  Out48 : Outport  Port=48
  Out49 : Outport  Port=49
  Out50 : Outport  Port=50
  Out51 : Outport  Port=51
  Out52 : Outport  Port=52
  Out53 : Outport  Port=53
  Out54 : Outport  Port=54
  Out55 : Outport  Port=55
  Out56 : Outport  Port=56
  Out57 : Outport  Port=57
  Out58 : Outport  Port=58
  Out59 : Outport  Port=59
  Out60 : Outport  Port=60
  Out61 : Outport  Port=61
  Out62 : Outport  Port=62
  Out63 : Outport  Port=63
  Out64 : Outport  Port=64
  wires:
  [Valido] -> Expression1/2
  Relational/1 -> Expression1/1
  [Dato] -> Delay4/1
  [Contador] -> Relational/1
  Constant19/1 -> Relational/2
  Expression1/1 -> Delay4/2
  Delay4/1 -> Out1/1
  [Valido] -> Expression2/2
  Relational1/1 -> Expression2/1
  [Dato] -> Delay1/1
  [Contador] -> Relational1/1
  Constant1/1 -> Relational1/2
  Expression2/1 -> Delay1/2
  Delay1/1 -> Out2/1
  [Valido] -> Expression3/2
  Relational2/1 -> Expression3/1
  [Dato] -> Delay2/1
  [Contador] -> Relational2/1
  Constant2/1 -> Relational2/2
  Expression3/1 -> Delay2/2
  Delay2/1 -> Out3/1
  [Valido] -> Expression4/2
  Relational3/1 -> Expression4/1
  [Dato] -> Delay3/1
  [Contador] -> Relational3/1
  Constant3/1 -> Relational3/2
  Expression4/1 -> Delay3/2
  Delay3/1 -> Out4/1
  [Valido] -> Expression5/2
  Relational4/1 -> Expression5/1
  [Dato] -> Delay8/1
  [Contador] -> Relational4/1
  Constant5/1 -> Relational4/2
  Expression5/1 -> Delay8/2
  Delay8/1 -> Out5/1
  [Valido] -> Expression6/2
  Relational5/1 -> Expression6/1
  [Dato] -> Delay5/1
  [Contador] -> Relational5/1
  Constant4/1 -> Relational5/2
  Expression6/1 -> Delay5/2
  Delay5/1 -> Out6/1
  [Valido] -> Expression7/2
  Relational6/1 -> Expression7/1
  [Dato] -> Delay6/1
  [Contador] -> Relational6/1
  Constant6/1 -> Relational6/2
  Expression7/1 -> Delay6/2
  Delay6/1 -> Out7/1
  [Valido] -> Expression8/2
  Relational7/1 -> Expression8/1
  [Dato] -> Delay7/1
  [Contador] -> Relational7/1
  Constant7/1 -> Relational7/2
  Expression8/1 -> Delay7/2
  Delay7/1 -> Out8/1
  [Valido] -> Expression9/2
  Relational8/1 -> Expression9/1
  [Dato] -> Delay12/1
  [Contador] -> Relational8/1
  Constant9/1 -> Relational8/2
  Expression9/1 -> Delay12/2
  Delay12/1 -> Out9/1
  [Valido] -> Expression10/2
  Relational9/1 -> Expression10/1
  [Dato] -> Delay9/1
  [Contador] -> Relational9/1
  Constant8/1 -> Relational9/2
  Expression10/1 -> Delay9/2
  Delay9/1 -> Out10/1
  [Valido] -> Expression11/2
  Relational10/1 -> Expression11/1
  [Dato] -> Delay10/1
  [Contador] -> Relational10/1
  Constant10/1 -> Relational10/2
  Expression11/1 -> Delay10/2
  Delay10/1 -> Out11/1
  [Valido] -> Expression12/2
  Relational11/1 -> Expression12/1
  [Dato] -> Delay11/1
  [Contador] -> Relational11/1
  Constant11/1 -> Relational11/2
  Expression12/1 -> Delay11/2
  Delay11/1 -> Out12/1
  [Valido] -> Expression13/2
  Relational12/1 -> Expression13/1
  [Dato] -> Delay16/1
  [Contador] -> Relational12/1
  Constant13/1 -> Relational12/2
  Expression13/1 -> Delay16/2
  Delay16/1 -> Out13/1
  [Valido] -> Expression14/2
  Relational13/1 -> Expression14/1
  [Dato] -> Delay13/1
  [Contador] -> Relational13/1
  Constant12/1 -> Relational13/2
  Expression14/1 -> Delay13/2
  Delay13/1 -> Out14/1
  [Valido] -> Expression15/2
  Relational14/1 -> Expression15/1
  [Dato] -> Delay14/1
  [Contador] -> Relational14/1
  Constant14/1 -> Relational14/2
  Expression15/1 -> Delay14/2
  Delay14/1 -> Out15/1
  [Valido] -> Expression16/2
  Relational15/1 -> Expression16/1
  [Dato] -> Delay15/1
  [Contador] -> Relational15/1
  Constant15/1 -> Relational15/2
  Expression16/1 -> Delay15/2
  Delay15/1 -> Out16/1
  [Valido] -> Expression17/2
  Relational16/1 -> Expression17/1
  [Dato] -> Delay27/1
  [Contador] -> Relational16/1
  Constant24/1 -> Relational16/2
  Delay27/1 -> Out17/1
  [Valido] -> Expression25/2
  Relational17/1 -> Expression25/1
  [Dato] -> Delay17/1
  [Contador] -> Relational17/1
  Constant16/1 -> Relational17/2
  Expression25/1 -> Delay17/2
  Delay17/1 -> Out18/1
  [Valido] -> Expression26/2
  Relational24/1 -> Expression26/1
  [Dato] -> Delay25/1
  [Contador] -> Relational24/1
  Constant25/1 -> Relational24/2
  Expression26/1 -> Delay25/2
  Delay25/1 -> Out19/1
  [Valido] -> Expression27/2
  Relational25/1 -> Expression27/1
  [Dato] -> Delay26/1
  [Contador] -> Relational25/1
  Constant26/1 -> Relational25/2
  Expression27/1 -> Delay26/2
  Delay26/1 -> Out20/1
  [Valido] -> Expression28/2
  Relational26/1 -> Expression28/1
  [Dato] -> Delay31/1
  [Contador] -> Relational26/1
  Constant28/1 -> Relational26/2
  Expression28/1 -> Delay31/2
  Delay31/1 -> Out21/1
  [Valido] -> Expression29/2
  Relational27/1 -> Expression29/1
  [Dato] -> Delay28/1
  [Contador] -> Relational27/1
  Constant27/1 -> Relational27/2
  Expression29/1 -> Delay28/2
  Delay28/1 -> Out22/1
  [Valido] -> Expression30/2
  Relational28/1 -> Expression30/1
  [Dato] -> Delay29/1
  [Contador] -> Relational28/1
  Constant29/1 -> Relational28/2
  Expression30/1 -> Delay29/2
  Delay29/1 -> Out23/1
  [Valido] -> Expression31/2
  Relational29/1 -> Expression31/1
  [Dato] -> Delay30/1
  [Contador] -> Relational29/1
  Constant30/1 -> Relational29/2
  Expression31/1 -> Delay30/2
  Delay30/1 -> Out24/1
  [Valido] -> Expression32/2
  Relational30/1 -> Expression32/1
  [Dato] -> Delay20/1
  [Contador] -> Relational30/1
  Constant32/1 -> Relational30/2
  Expression32/1 -> Delay20/2
  Delay20/1 -> Out25/1
  [Valido] -> Expression18/2
  Relational31/1 -> Expression18/1
  [Dato] -> Delay32/1
  [Contador] -> Relational31/1
  Constant31/1 -> Relational31/2
  Expression18/1 -> Delay32/2
  Delay32/1 -> Out26/1
  [Valido] -> Expression19/2
  Relational18/1 -> Expression19/1
  [Dato] -> Delay18/1
  [Contador] -> Relational18/1
  Constant17/1 -> Relational18/2
  Expression19/1 -> Delay18/2
  Delay18/1 -> Out27/1
  [Valido] -> Expression20/2
  Relational19/1 -> Expression20/1
  [Dato] -> Delay19/1
  [Contador] -> Relational19/1
  Constant18/1 -> Relational19/2
  Expression20/1 -> Delay19/2
  Delay19/1 -> Out28/1
  [Valido] -> Expression21/2
  Relational20/1 -> Expression21/1
  [Dato] -> Delay24/1
  [Contador] -> Relational20/1
  Constant21/1 -> Relational20/2
  Expression21/1 -> Delay24/2
  Delay24/1 -> Out29/1
  [Valido] -> Expression22/2
  Relational21/1 -> Expression22/1
  [Dato] -> Delay21/1
  [Contador] -> Relational21/1
  Constant20/1 -> Relational21/2
  Expression22/1 -> Delay21/2
  Delay21/1 -> Out30/1
  [Valido] -> Expression23/2
  Relational22/1 -> Expression23/1
  [Dato] -> Delay22/1
  [Contador] -> Relational22/1
  Constant22/1 -> Relational22/2
  Expression23/1 -> Delay22/2
  Delay22/1 -> Out31/1
  [Valido] -> Expression24/2
  Relational23/1 -> Expression24/1
  [Dato] -> Delay23/1
  [Contador] -> Relational23/1
  Constant23/1 -> Relational23/2
  Expression24/1 -> Delay23/2
  Delay23/1 -> Out32/1
  [Valido] -> Expression33/2
  Relational32/1 -> Expression33/1
  [Dato] -> Delay59/1
  [Contador] -> Relational32/1
  Constant43/1 -> Relational32/2
  Expression33/1 -> Delay59/2
  Delay59/1 -> Out33/1
  [Valido] -> Expression44/2
  Relational33/1 -> Expression44/1
  [Dato] -> Delay33/1
  [Contador] -> Relational33/1
  Constant33/1 -> Relational33/2
  Expression44/1 -> Delay33/2
  Delay33/1 -> Out34/1
  [Valido] -> Expression55/2
  Relational44/1 -> Expression55/1
  [Dato] -> Delay44/1
  [Contador] -> Relational44/1
  Constant44/1 -> Relational44/2
  Expression55/1 -> Delay44/2
  Delay44/1 -> Out35/1
  [Valido] -> Expression59/2
  Relational55/1 -> Expression59/1
  [Dato] -> Delay55/1
  [Contador] -> Relational55/1
  Constant55/1 -> Relational55/2
  Expression59/1 -> Delay55/2
  Delay55/1 -> Out36/1
  [Valido] -> Expression60/2
  Relational58/1 -> Expression60/1
  [Dato] -> Delay63/1
  [Contador] -> Relational58/1
  Constant60/1 -> Relational58/2
  Expression60/1 -> Delay63/2
  Delay63/1 -> Out37/1
  [Valido] -> Expression61/2
  Relational59/1 -> Expression61/1
  [Dato] -> Delay60/1
  [Contador] -> Relational59/1
  Constant59/1 -> Relational59/2
  Expression61/1 -> Delay60/2
  Delay60/1 -> Out38/1
  [Valido] -> Expression62/2
  Relational60/1 -> Expression62/1
  [Dato] -> Delay61/1
  [Contador] -> Relational60/1
  Constant61/1 -> Relational60/2
  Expression62/1 -> Delay61/2
  Delay61/1 -> Out39/1
  [Valido] -> Expression63/2
  Relational61/1 -> Expression63/1
  [Dato] -> Delay62/1
  [Contador] -> Relational61/1
  Constant62/1 -> Relational61/2
  Expression63/1 -> Delay62/2
  Delay62/1 -> Out40/1
  [Valido] -> Expression64/2
  Relational62/1 -> Expression64/1
  [Dato] -> Delay36/1
  [Contador] -> Relational62/1
  Constant64/1 -> Relational62/2
  Expression64/1 -> Delay36/2
  Delay36/1 -> Out41/1
  [Valido] -> Expression34/2
  Relational63/1 -> Expression34/1
  [Dato] -> Delay64/1
  [Contador] -> Relational63/1
  Constant63/1 -> Relational63/2
  Expression34/1 -> Delay64/2
  Delay64/1 -> Out42/1
  [Valido] -> Expression35/2
  Relational34/1 -> Expression35/1
  [Dato] -> Delay34/1
  [Contador] -> Relational34/1
  Constant34/1 -> Relational34/2
  Expression35/1 -> Delay34/2
  Delay34/1 -> Out43/1
  [Valido] -> Expression36/2
  Relational35/1 -> Expression36/1
  [Dato] -> Delay35/1
  [Contador] -> Relational35/1
  Constant35/1 -> Relational35/2
  Expression36/1 -> Delay35/2
  Delay35/1 -> Out44/1
  [Valido] -> Expression37/2
  Relational36/1 -> Expression37/1
  [Dato] -> Delay40/1
  [Contador] -> Relational36/1
  Constant37/1 -> Relational36/2
  Expression37/1 -> Delay40/2
  Delay40/1 -> Out45/1
  [Valido] -> Expression38/2
  Relational37/1 -> Expression38/1
  [Dato] -> Delay37/1
  [Contador] -> Relational37/1
  Constant36/1 -> Relational37/2
  Expression38/1 -> Delay37/2
  Delay37/1 -> Out46/1
  [Valido] -> Expression39/2
  Relational38/1 -> Expression39/1
  [Dato] -> Delay38/1
  [Contador] -> Relational38/1
  Constant38/1 -> Relational38/2
  Expression39/1 -> Delay38/2
  Delay38/1 -> Out47/1
  [Valido] -> Expression40/2
  Relational39/1 -> Expression40/1
  [Dato] -> Delay39/1
  [Contador] -> Relational39/1
  Constant39/1 -> Relational39/2
  Expression40/1 -> Delay39/2
  Delay39/1 -> Out48/1
  [Valido] -> Expression41/2
  Relational40/1 -> Expression41/1
  [Dato] -> Delay52/1
  [Contador] -> Relational40/1
  Constant49/1 -> Relational40/2
  Expression41/1 -> Delay52/2
  Delay52/1 -> Out49/1
  [Valido] -> Expression50/2
  Relational41/1 -> Expression50/1
  [Dato] -> Delay41/1
  [Contador] -> Relational41/1
  Constant40/1 -> Relational41/2
  Expression50/1 -> Delay41/2
  Delay41/1 -> Out50/1
  [Valido] -> Expression51/2
  Relational49/1 -> Expression51/1
  [Dato] -> Delay50/1
  [Contador] -> Relational49/1
  Constant50/1 -> Relational49/2
  Expression51/1 -> Delay50/2
  Delay50/1 -> Out51/1
  [Valido] -> Expression52/2
  Relational50/1 -> Expression52/1
  [Dato] -> Delay51/1
  [Contador] -> Relational50/1
  Constant51/1 -> Relational50/2
  Expression52/1 -> Delay51/2
  Delay51/1 -> Out52/1
  [Valido] -> Expression53/2
  Relational51/1 -> Expression53/1
  [Dato] -> Delay57/1
  [Contador] -> Relational51/1
  Constant53/1 -> Relational51/2
  Expression53/1 -> Delay57/2
  Delay57/1 -> Out53/1
  [Valido] -> Expression54/2
  Relational52/1 -> Expression54/1
  [Dato] -> Delay53/1
  [Contador] -> Relational52/1
  Constant52/1 -> Relational52/2
  Expression54/1 -> Delay53/2
  Delay53/1 -> Out54/1
  [Valido] -> Expression56/2
  Relational53/1 -> Expression56/1
  [Dato] -> Delay54/1
  [Contador] -> Relational53/1
  Constant54/1 -> Relational53/2
  Expression56/1 -> Delay54/2
  Delay54/1 -> Out55/1
  [Valido] -> Expression57/2
  Relational54/1 -> Expression57/1
  [Dato] -> Delay56/1
  [Contador] -> Relational54/1
  Constant56/1 -> Relational54/2
  Expression57/1 -> Delay56/2
  Delay56/1 -> Out56/1
  [Valido] -> Expression58/2
  Relational56/1 -> Expression58/1
  [Dato] -> Delay45/1
  [Contador] -> Relational56/1
  Constant58/1 -> Relational56/2
  Expression58/1 -> Delay45/2
  Delay45/1 -> Out57/1
  [Valido] -> Expression42/2
  Relational57/1 -> Expression42/1
  [Dato] -> Delay58/1
  [Contador] -> Relational57/1
  Constant57/1 -> Relational57/2
  Expression42/1 -> Delay58/2
  Delay58/1 -> Out58/1
  [Valido] -> Expression43/2
  Relational42/1 -> Expression43/1
  [Dato] -> Delay42/1
  [Contador] -> Relational42/1
  Constant41/1 -> Relational42/2
  Expression43/1 -> Delay42/2
  Delay42/1 -> Out59/1
  [Valido] -> Expression45/2
  Relational43/1 -> Expression45/1
  [Dato] -> Delay43/1
  [Contador] -> Relational43/1
  Constant42/1 -> Relational43/2
  Expression45/1 -> Delay43/2
  Delay43/1 -> Out60/1
  [Valido] -> Expression46/2
  Relational45/1 -> Expression46/1
  [Dato] -> Delay49/1
  [Contador] -> Relational45/1
  Constant46/1 -> Relational45/2
  Expression46/1 -> Delay49/2
  Delay49/1 -> Out61/1
  [Valido] -> Expression47/2
  Relational46/1 -> Expression47/1
  [Dato] -> Delay46/1
  [Contador] -> Relational46/1
  Constant45/1 -> Relational46/2
  Expression47/1 -> Delay46/2
  Delay46/1 -> Out62/1
  [Valido] -> Expression48/2
  Relational47/1 -> Expression48/1
  [Dato] -> Delay47/1
  [Contador] -> Relational47/1
  Constant47/1 -> Relational47/2
  Expression48/1 -> Delay47/2
  Delay47/1 -> Out63/1
  [Valido] -> Expression49/2
  Relational48/1 -> Expression49/1
  [Dato] -> Delay48/1
  [Contador] -> Relational48/1
  Constant48/1 -> Relational48/2
  Expression49/1 -> Delay48/2
  Delay48/1 -> Out64/1
  Expression17/1 -> Delay27/2
